simulink model "test_mdl"  (R2018a)
settings: Solver=VariableStepAuto  StartTime=0.0  StopTime=10.0  RelTol=1e-3
(part 5 of 8)

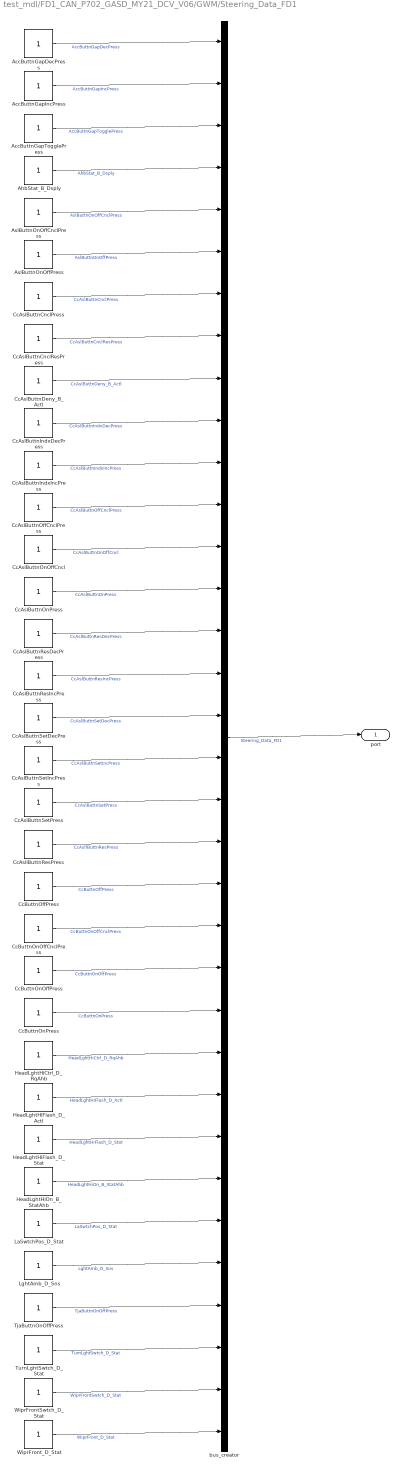
== system test_mdl/FD1_CAN_P702_GASD_MY21_DCV_V06/GWM/Steering_Data_FD1 ==
  AccButtnGapDecPress : Constant
  AccButtnGapIncPress : Constant
  AccButtnGapTogglePress : Constant
  AhbStat_B_Dsply : Constant
  AslButtnOnOffCnclPress : Constant
  AslButtnOnOffPress : Constant
  CcAslButtnCnclPress : Constant
  CcAslButtnCnclResPress : Constant
  CcAslButtnDeny_B_Actl : Constant
  CcAslButtnIndxDecPress : Constant
  CcAslButtnIndxIncPress : Constant
  CcAslButtnOffCnclPress : Constant
  CcAslButtnOnOffCncl : Constant
  CcAslButtnOnPress : Constant
  CcAslButtnResDecPress : Constant
  CcAslButtnResIncPress : Constant
  CcAslButtnSetDecPress : Constant
  CcAslButtnSetIncPress : Constant
  CcAslButtnSetPress : Constant
  CcAsllButtnResPress : Constant
  CcButtnOffPress : Constant
  CcButtnOnOffCnclPress : Constant
  CcButtnOnOffPress : Constant
  CcButtnOnPress : Constant
  HeadLghtHiCtrl_D_RqAhb : Constant
  HeadLghtHiFlash_D_Actl : Constant
  HeadLghtHiFlash_D_Stat : Constant
  HeadLghtHiOn_B_StatAhb : Constant
  LaSwtchPos_D_Stat : Constant
  LghtAmb_D_Sns : Constant
  TjaButtnOnOffPress : Constant
  TurnLghtSwtch_D_Stat : Constant
  WiprFrontSwtch_D_Stat : Constant
  WiprFront_D_Stat : Constant
  bus_creator : BusCreator  Inputs=34
  port : Outport
  wires:
  bus_creator/1 -> port/1  "Steering_Data_FD1"
  AccButtnGapDecPress/1 -> bus_creator/1  "AccButtnGapDecPress"
  AccButtnGapIncPress/1 -> bus_creator/2  "AccButtnGapIncPress"
  AccButtnGapTogglePress/1 -> bus_creator/3  "AccButtnGapTogglePress"
  AhbStat_B_Dsply/1 -> bus_creator/4  "AhbStat_B_Dsply"
  AslButtnOnOffCnclPress/1 -> bus_creator/5  "AslButtnOnOffCnclPress"
  AslButtnOnOffPress/1 -> bus_creator/6  "AslButtnOnOffPress"
  CcAslButtnCnclPress/1 -> bus_creator/7  "CcAslButtnCnclPress"
  CcAslButtnCnclResPress/1 -> bus_creator/8  "CcAslButtnCnclResPress"
  CcAslButtnDeny_B_Actl/1 -> bus_creator/9  "CcAslButtnDeny_B_Actl"
  CcAslButtnIndxDecPress/1 -> bus_creator/10  "CcAslButtnIndxDecPress"
  CcAslButtnIndxIncPress/1 -> bus_creator/11  "CcAslButtnIndxIncPress"
  CcAslButtnOffCnclPress/1 -> bus_creator/12  "CcAslButtnOffCnclPress"
  CcAslButtnOnOffCncl/1 -> bus_creator/13  "CcAslButtnOnOffCncl"
  CcAslButtnOnPress/1 -> bus_creator/14  "CcAslButtnOnPress"
  CcAslButtnResDecPress/1 -> bus_creator/15  "CcAslButtnResDecPress"
  CcAslButtnResIncPress/1 -> bus_creator/16  "CcAslButtnResIncPress"
  CcAslButtnSetDecPress/1 -> bus_creator/17  "CcAslButtnSetDecPress"
  CcAslButtnSetIncPress/1 -> bus_creator/18  "CcAslButtnSetIncPress"
  CcAslButtnSetPress/1 -> bus_creator/19  "CcAslButtnSetPress"
  CcAsllButtnResPress/1 -> bus_creator/20  "CcAsllButtnResPress"
  CcButtnOffPress/1 -> bus_creator/21  "CcButtnOffPress"
  CcButtnOnOffCnclPress/1 -> bus_creator/22  "CcButtnOnOffCnclPress"
  CcButtnOnOffPress/1 -> bus_creator/23  "CcButtnOnOffPress"
  CcButtnOnPress/1 -> bus_creator/24  "CcButtnOnPress"
  HeadLghtHiCtrl_D_RqAhb/1 -> bus_creator/25  "HeadLghtHiCtrl_D_RqAhb"
  HeadLghtHiFlash_D_Actl/1 -> bus_creator/26  "HeadLghtHiFlash_D_Actl"
  HeadLghtHiFlash_D_Stat/1 -> bus_creator/27  "HeadLghtHiFlash_D_Stat"
  HeadLghtHiOn_B_StatAhb/1 -> bus_creator/28  "HeadLghtHiOn_B_StatAhb"
  LaSwtchPos_D_Stat/1 -> bus_creator/29  "LaSwtchPos_D_Stat"
  LghtAmb_D_Sns/1 -> bus_creator/30  "LghtAmb_D_Sns"
  TjaButtnOnOffPress/1 -> bus_creator/31  "TjaButtnOnOffPress"
  TurnLghtSwtch_D_Stat/1 -> bus_creator/32  "TurnLghtSwtch_D_Stat"
  WiprFrontSwtch_D_Stat/1 -> bus_creator/33  "WiprFrontSwtch_D_Stat"
  WiprFront_D_Stat/1 -> bus_creator/34  "WiprFront_D_Stat"

== system test_mdl/FD1_CAN_P702_GASD_MY21_DCV_V06/GWM/Steering_Wheel_Data2_FD1 ==
  SelDrvMdeDec_B_RqDrv : Constant
  SelDrvMdeInc_B_RqDrv : Constant
  SelDrvMdeSwtch_D_Stat4 : Constant
  SteEffortInc_B_RqDrv : Constant
  SteWhlSwtchBack_B_Stat : Constant
  SteWhlSwtchDown_B_Stat : Constant
  SteWhlSwtchHome_B_Stat : Constant
  SteWhlSwtchHud_B_Stat : Constant
  SteWhlSwtchInfo_B_Stat : Constant
  SteWhlSwtchIod_B_Stat : Constant
  SteWhlSwtchLeft_B_Stat : Constant
  SteWhlSwtchMed_B_Stat : Constant
  SteWhlSwtchMenu_B_Stat : Constant
  SteWhlSwtchNav_B_Stat : Constant
  SteWhlSwtchOk_B_Stat : Constant
  SteWhlSwtchPhon_B_Stat : Constant
  SteWhlSwtchRght_B_Stat : Constant
  SteWhlSwtchSet_B_Stat : Constant
  SteWhlSwtchUp_B_Stat : Constant
  SteWhlSwtchView_B_Stat : Constant
  SuspDampInc_B_RqDrv : Constant
  bus_creator : BusCreator  Inputs=21
  port : Outport
  wires:
  bus_creator/1 -> port/1  "Steering_Wheel_Data2_FD1"
  SelDrvMdeDec_B_RqDrv/1 -> bus_creator/1  "SelDrvMdeDec_B_RqDrv"
  SelDrvMdeInc_B_RqDrv/1 -> bus_creator/2  "SelDrvMdeInc_B_RqDrv"
  SelDrvMdeSwtch_D_Stat4/1 -> bus_creator/3  "SelDrvMdeSwtch_D_Stat4"
  SteEffortInc_B_RqDrv/1 -> bus_creator/4  "SteEffortInc_B_RqDrv"
  SteWhlSwtchBack_B_Stat/1 -> bus_creator/5  "SteWhlSwtchBack_B_Stat"
  SteWhlSwtchDown_B_Stat/1 -> bus_creator/6  "SteWhlSwtchDown_B_Stat"
  SteWhlSwtchHome_B_Stat/1 -> bus_creator/7  "SteWhlSwtchHome_B_Stat"
  SteWhlSwtchHud_B_Stat/1 -> bus_creator/8  "SteWhlSwtchHud_B_Stat"
  SteWhlSwtchInfo_B_Stat/1 -> bus_creator/9  "SteWhlSwtchInfo_B_Stat"
  SteWhlSwtchIod_B_Stat/1 -> bus_creator/10  "SteWhlSwtchIod_B_Stat"
  SteWhlSwtchLeft_B_Stat/1 -> bus_creator/11  "SteWhlSwtchLeft_B_Stat"
  SteWhlSwtchMed_B_Stat/1 -> bus_creator/12  "SteWhlSwtchMed_B_Stat"
  SteWhlSwtchMenu_B_Stat/1 -> bus_creator/13  "SteWhlSwtchMenu_B_Stat"
  SteWhlSwtchNav_B_Stat/1 -> bus_creator/14  "SteWhlSwtchNav_B_Stat"
  SteWhlSwtchOk_B_Stat/1 -> bus_creator/15  "SteWhlSwtchOk_B_Stat"
  SteWhlSwtchPhon_B_Stat/1 -> bus_creator/16  "SteWhlSwtchPhon_B_Stat"
  SteWhlSwtchRght_B_Stat/1 -> bus_creator/17  "SteWhlSwtchRght_B_Stat"
  SteWhlSwtchSet_B_Stat/1 -> bus_creator/18  "SteWhlSwtchSet_B_Stat"
  SteWhlSwtchUp_B_Stat/1 -> bus_creator/19  "SteWhlSwtchUp_B_Stat"
  SteWhlSwtchView_B_Stat/1 -> bus_creator/20  "SteWhlSwtchView_B_Stat"
  SuspDampInc_B_RqDrv/1 -> bus_creator/21  "SuspDampInc_B_RqDrv"

== system test_mdl/FD1_CAN_P702_GASD_MY21_DCV_V06/GWM/TCU_Send_Signals_FD1 ==
  EmgcyCallMute_D_Stat : Constant
  OfbChrgSetSync_D_Rq : Constant
  TelematicsSrvc_D_St : Constant
  bus_creator : BusCreator  Inputs=3
  port : Outport
  wires:
  bus_creator/1 -> port/1  "TCU_Send_Signals_FD1"
  EmgcyCallMute_D_Stat/1 -> bus_creator/1  "EmgcyCallMute_D_Stat"
  OfbChrgSetSync_D_Rq/1 -> bus_creator/2  "OfbChrgSetSync_D_Rq"
  TelematicsSrvc_D_St/1 -> bus_creator/3  "TelematicsSrvc_D_St"

== system test_mdl/FD1_CAN_P702_GASD_MY21_DCV_V06/GWM/TesterPhysicalReqVDM_FD1 ==
  TesterPhysicalReqVDM : Constant
  bus_creator : BusCreator  Inputs=1
  port : Outport
  wires:
  bus_creator/1 -> port/1  "TesterPhysicalReqVDM_FD1"
  TesterPhysicalReqVDM/1 -> bus_creator/1  "TesterPhysicalReqVDM"

== system test_mdl/FD1_CAN_P702_GASD_MY21_DCV_V06/GWM/TesterPhysicalResGWM_FD1 ==
  TesterPhysicalResGWM_F1 : Constant
  bus_creator : BusCreator  Inputs=1
  port : Outport
  wires:
  bus_creator/1 -> port/1  "TesterPhysicalResGWM_FD1"
  TesterPhysicalResGWM_F1/1 -> bus_creator/1  "TesterPhysicalResGWM_F1"

== system test_mdl/FD1_CAN_P702_GASD_MY21_DCV_V06/GWM/Tire_Pressure_Data_FD1 ==
  Tire_Press_LF_Data : Constant
  Tire_Press_LR_OLR_Data : Constant
  Tire_Press_RF_Data : Constant
  Tire_Press_RR_ORR_Data : Constant
  bus_creator : BusCreator  Inputs=4
  port : Outport
  wires:
  bus_creator/1 -> port/1  "Tire_Pressure_Data_FD1"
  Tire_Press_LF_Data/1 -> bus_creator/1  "Tire_Press_LF_Data"
  Tire_Press_LR_OLR_Data/1 -> bus_creator/2  "Tire_Press_LR_OLR_Data"
  Tire_Press_RF_Data/1 -> bus_creator/3  "Tire_Press_RF_Data"
  Tire_Press_RR_ORR_Data/1 -> bus_creator/4  "Tire_Press_RR_ORR_Data"

== system test_mdl/FD1_CAN_P702_GASD_MY21_DCV_V06/GWM/TrailerAid_Data3_FD1 ==
  TrlrAidEnbl_D2_Rq : Constant
  TrlrAidSetup_D2_Rq : Constant
  TrlrAnOffstDir_D_Mem : Constant
  TrlrAnOffst_An_Mem : Constant
  TrlrAxleToBmpr_L_Actl : Constant
  TrlrBallToBmpr_L_Actl : Constant
  TrlrIdType_D_Stat : Constant
  TrlrId_No_Actl : Constant
  TrlrRvrseCancl_B_Rq : Constant
  TrlrTrgtOffst_L_Actl : Constant
  TrlrTrgtPtrnId_No_Mem : Constant
  TrlrTrgtToBmpr_L_Actl : Constant
  bus_creator : BusCreator  Inputs=12
  port : Outport
  wires:
  bus_creator/1 -> port/1  "TrailerAid_Data3_FD1"
  TrlrAidEnbl_D2_Rq/1 -> bus_creator/1  "TrlrAidEnbl_D2_Rq"
  TrlrAidSetup_D2_Rq/1 -> bus_creator/2  "TrlrAidSetup_D2_Rq"
  TrlrAnOffstDir_D_Mem/1 -> bus_creator/3  "TrlrAnOffstDir_D_Mem"
  TrlrAnOffst_An_Mem/1 -> bus_creator/4  "TrlrAnOffst_An_Mem"
  TrlrAxleToBmpr_L_Actl/1 -> bus_creator/5  "TrlrAxleToBmpr_L_Actl"
  TrlrBallToBmpr_L_Actl/1 -> bus_creator/6  "TrlrBallToBmpr_L_Actl"
  TrlrIdType_D_Stat/1 -> bus_creator/7  "TrlrIdType_D_Stat"
  TrlrId_No_Actl/1 -> bus_creator/8  "TrlrId_No_Actl"
  TrlrRvrseCancl_B_Rq/1 -> bus_creator/9  "TrlrRvrseCancl_B_Rq"
  TrlrTrgtOffst_L_Actl/1 -> bus_creator/10  "TrlrTrgtOffst_L_Actl"
  TrlrTrgtPtrnId_No_Mem/1 -> bus_creator/11  "TrlrTrgtPtrnId_No_Mem"
  TrlrTrgtToBmpr_L_Actl/1 -> bus_creator/12  "TrlrTrgtToBmpr_L_Actl"

== system test_mdl/FD1_CAN_P702_GASD_MY21_DCV_V06/GWM/TrailerAid_Data_FD1 ==
  TrailCtlSwtch_B_Stat2 : Constant
  TrlBrkInitOut_D_Rq : Constant
  bus_creator : BusCreator  Inputs=2
  port : Outport
  wires:
  bus_creator/1 -> port/1  "TrailerAid_Data_FD1"
  TrailCtlSwtch_B_Stat2/1 -> bus_creator/1  "TrailCtlSwtch_B_Stat2"
  TrlBrkInitOut_D_Rq/1 -> bus_creator/2  "TrlBrkInitOut_D_Rq"

== system test_mdl/FD1_CAN_P702_GASD_MY21_DCV_V06/GWM/TrailerAid_Stat1_FD1 ==
  TrlrSnsId_No_Actl : Constant
  bus_creator : BusCreator  Inputs=1
  port : Outport
  wires:
  bus_creator/1 -> port/1  "TrailerAid_Stat1_FD1"
  TrlrSnsId_No_Actl/1 -> bus_creator/1  "TrlrSnsId_No_Actl"

== system test_mdl/FD1_CAN_P702_GASD_MY21_DCV_V06/GWM/TrailerAid_Stat2_FD1 ==
  TrlrHitYaw_AnRate_Actl : Constant
  TrlrHitchYaw_An_Actl : Constant
  TrlrHitchYaw_D_Stat : Constant
  TrlrYawWActl_D_Qf : Constant
  TrlrYaw_W_Actl : Constant
  bus_creator : BusCreator  Inputs=5
  port : Outport
  wires:
  bus_creator/1 -> port/1  "TrailerAid_Stat2_FD1"
  TrlrHitYaw_AnRate_Actl/1 -> bus_creator/1  "TrlrHitYaw_AnRate_Actl"
  TrlrHitchYaw_An_Actl/1 -> bus_creator/2  "TrlrHitchYaw_An_Actl"
  TrlrHitchYaw_D_Stat/1 -> bus_creator/3  "TrlrHitchYaw_D_Stat"
  TrlrYawWActl_D_Qf/1 -> bus_creator/4  "TrlrYawWActl_D_Qf"
  TrlrYaw_W_Actl/1 -> bus_creator/5  "TrlrYaw_W_Actl"

== system test_mdl/FD1_CAN_P702_GASD_MY21_DCV_V06/GWM/TrailerBrakeInfo_FD1 ==
  StopLamp_B_RqTrlrBrk : Constant
  TrlBrkInitOut_D_Stat : Constant
  TrlrBrkActCirct_B_Falt : Constant
  TrlrBrkActCnnct_B_Actl : Constant
  TrlrBrkCtl_B_Falt : Constant
  TrlrBrkDcnnt_B_Actl : Constant
  TrlrBrkDsply_B_Rq : Constant
  TrlrBrkGain_No_Actl : Constant
  TrlrBrkMde_D_Actl : Constant
  TrlrBrkOut_No_Dsply : Constant
  bus_creator : BusCreator  Inputs=10
  port : Outport
  wires:
  bus_creator/1 -> port/1  "TrailerBrakeInfo_FD1"
  StopLamp_B_RqTrlrBrk/1 -> bus_creator/1  "StopLamp_B_RqTrlrBrk"
  TrlBrkInitOut_D_Stat/1 -> bus_creator/2  "TrlBrkInitOut_D_Stat"
  TrlrBrkActCirct_B_Falt/1 -> bus_creator/3  "TrlrBrkActCirct_B_Falt"
  TrlrBrkActCnnct_B_Actl/1 -> bus_creator/4  "TrlrBrkActCnnct_B_Actl"
  TrlrBrkCtl_B_Falt/1 -> bus_creator/5  "TrlrBrkCtl_B_Falt"
  TrlrBrkDcnnt_B_Actl/1 -> bus_creator/6  "TrlrBrkDcnnt_B_Actl"
  TrlrBrkDsply_B_Rq/1 -> bus_creator/7  "TrlrBrkDsply_B_Rq"
  TrlrBrkGain_No_Actl/1 -> bus_creator/8  "TrlrBrkGain_No_Actl"
  TrlrBrkMde_D_Actl/1 -> bus_creator/9  "TrlrBrkMde_D_Actl"
  TrlrBrkOut_No_Dsply/1 -> bus_creator/10  "TrlrBrkOut_No_Dsply"

== system test_mdl/FD1_CAN_P702_GASD_MY21_DCV_V06/GWM/TrailerInfo_2_FD1 ==
  TrlrAidCtl_U_RqDrv : Constant
  TrlrAidSwtch_D_RqDrv : Constant
  bus_creator : BusCreator  Inputs=2
  port : Outport
  wires:
  bus_creator/1 -> port/1  "TrailerInfo_2_FD1"
  TrlrAidCtl_U_RqDrv/1 -> bus_creator/1  "TrlrAidCtl_U_RqDrv"
  TrlrAidSwtch_D_RqDrv/1 -> bus_creator/2  "TrlrAidSwtch_D_RqDrv"

== system test_mdl/FD1_CAN_P702_GASD_MY21_DCV_V06/GWM/TrailerInfo_FD1 ==
  ParkLampTrlrOut_B_Stat : Constant
  StopLampTrlrOut_B_Stat : Constant
  TrlrBattChrg_D_Stat : Constant
  TrlrLampCnnct_B_Actl : Constant
  TrlrLampCtl_D_Stat : Constant
  TurnLampTrlrRl_B_Stat : Constant
  TurnLampTrlrRr_B_Stat : Constant
  bus_creator : BusCreator  Inputs=7
  port : Outport
  wires:
  bus_creator/1 -> port/1  "TrailerInfo_FD1"
  ParkLampTrlrOut_B_Stat/1 -> bus_creator/1  "ParkLampTrlrOut_B_Stat"
  StopLampTrlrOut_B_Stat/1 -> bus_creator/2  "StopLampTrlrOut_B_Stat"
  TrlrBattChrg_D_Stat/1 -> bus_creator/3  "TrlrBattChrg_D_Stat"
  TrlrLampCnnct_B_Actl/1 -> bus_creator/4  "TrlrLampCnnct_B_Actl"
  TrlrLampCtl_D_Stat/1 -> bus_creator/5  "TrlrLampCtl_D_Stat"
  TurnLampTrlrRl_B_Stat/1 -> bus_creator/6  "TurnLampTrlrRl_B_Stat"
  TurnLampTrlrRr_B_Stat/1 -> bus_creator/7  "TurnLampTrlrRr_B_Stat"

== system test_mdl/FD1_CAN_P702_GASD_MY21_DCV_V06/GWM/Voltage_Power_Data2_FD1 ==
  CoolFanDcdc_D_Rq : Constant
  DcdcClntFlw_D_Rq : Constant
  bus_creator : BusCreator  Inputs=2
  port : Outport
  wires:
  bus_creator/1 -> port/1  "Voltage_Power_Data2_FD1"
  CoolFanDcdc_D_Rq/1 -> bus_creator/1  "CoolFanDcdc_D_Rq"
  DcdcClntFlw_D_Rq/1 -> bus_creator/2  "DcdcClntFlw_D_Rq"

== system test_mdl/FD1_CAN_P702_GASD_MY21_DCV_V06/GWM/Yaw_Data_FD1 ==
  VehRolWActl_D_Qf : Constant
  VehRol_W_Actl : Constant
  VehRollYawW_No_Cs : Constant
  VehRollYaw_No_Cnt : Constant
  VehYawWActl_D_Qf : Constant
  VehYaw_W_Actl : Constant
  bus_creator : BusCreator  Inputs=6
  port : Outport
  wires:
  bus_creator/1 -> port/1  "Yaw_Data_FD1"
  VehRolWActl_D_Qf/1 -> bus_creator/1  "VehRolWActl_D_Qf"
  VehRol_W_Actl/1 -> bus_creator/2  "VehRol_W_Actl"
  VehRollYawW_No_Cs/1 -> bus_creator/3  "VehRollYawW_No_Cs"
  VehRollYaw_No_Cnt/1 -> bus_creator/4  "VehRollYaw_No_Cnt"
  VehYawWActl_D_Qf/1 -> bus_creator/5  "VehYawWActl_D_Qf"
  VehYaw_W_Actl/1 -> bus_creator/6  "VehYaw_W_Actl"

== system test_mdl/FD1_CAN_P702_GASD_MY21_DCV_V06/IPMA_ADAS/ACCDATA ==
  AccAutoResum_D_Rq : Constant
  AccBrkDecel_B_Rq : Constant
  AccBrkPrchg_B_Rq : Constant
  AccBrkPrkEl_B_Rq : Constant
  AccBrkPulse_B_Rq : Constant
  AccBrkTot_A_Rq : Constant
  AccCancl_B_Rq : Constant
  AccDeny_B_Rq : Constant
  AccPrpl_A_Pred : Constant
  AccPrpl_A_Rq : Constant
  AccResumEnbl_B_Rq : Constant
  AccStopStat_B_Rq : Constant
  AccVeh_V_Trg : Constant
  CmbbDeny_B_Actl : Constant
  CmbbEngTqMn_B_Rq : Constant
  CmbbOvrrd_B_RqDrv : Constant
  Cmbb_B_Enbl : Constant
  bus_creator : BusCreator  Inputs=17
  port : Outport
  wires:
  bus_creator/1 -> port/1  "ACCDATA"
  AccAutoResum_D_Rq/1 -> bus_creator/1  "AccAutoResum_D_Rq"
  AccBrkDecel_B_Rq/1 -> bus_creator/2  "AccBrkDecel_B_Rq"
  AccBrkPrchg_B_Rq/1 -> bus_creator/3  "AccBrkPrchg_B_Rq"
  AccBrkPrkEl_B_Rq/1 -> bus_creator/4  "AccBrkPrkEl_B_Rq"
  AccBrkPulse_B_Rq/1 -> bus_creator/5  "AccBrkPulse_B_Rq"
  AccBrkTot_A_Rq/1 -> bus_creator/6  "AccBrkTot_A_Rq"
  AccCancl_B_Rq/1 -> bus_creator/7  "AccCancl_B_Rq"
  AccDeny_B_Rq/1 -> bus_creator/8  "AccDeny_B_Rq"
  AccPrpl_A_Pred/1 -> bus_creator/9  "AccPrpl_A_Pred"
  AccPrpl_A_Rq/1 -> bus_creator/10  "AccPrpl_A_Rq"
  AccResumEnbl_B_Rq/1 -> bus_creator/11  "AccResumEnbl_B_Rq"
  AccStopStat_B_Rq/1 -> bus_creator/12  "AccStopStat_B_Rq"
  AccVeh_V_Trg/1 -> bus_creator/13  "AccVeh_V_Trg"
  CmbbDeny_B_Actl/1 -> bus_creator/14  "CmbbDeny_B_Actl"
  CmbbEngTqMn_B_Rq/1 -> bus_creator/15  "CmbbEngTqMn_B_Rq"
  CmbbOvrrd_B_RqDrv/1 -> bus_creator/16  "CmbbOvrrd_B_RqDrv"
  Cmbb_B_Enbl/1 -> bus_creator/17  "Cmbb_B_Enbl"

== system test_mdl/FD1_CAN_P702_GASD_MY21_DCV_V06/IPMA_ADAS/ACCDATA_2 ==
  CmbbBaSens_D_Rq : Constant
  CmbbBrkDecel_A_Rq : Constant
  CmbbBrkDecel_B_Rq : Constant
  CmbbBrkDecel_No_Cnt : Constant
  CmbbBrkDecel_No_Cs : Constant
  CmbbBrkPrchg_D_Rq : Constant
  HudBlk1_B_Rq : Constant
  HudBlk2_B_Rq : Constant
  HudBlk3_B_Rq : Constant
  HudDsplyIntns_No_Actl : Constant
  HudFlashRate_D_Actl : Constant
  bus_creator : BusCreator  Inputs=11
  port : Outport
  wires:
  bus_creator/1 -> port/1  "ACCDATA_2"
  CmbbBaSens_D_Rq/1 -> bus_creator/1  "CmbbBaSens_D_Rq"
  CmbbBrkDecel_A_Rq/1 -> bus_creator/2  "CmbbBrkDecel_A_Rq"
  CmbbBrkDecel_B_Rq/1 -> bus_creator/3  "CmbbBrkDecel_B_Rq"
  CmbbBrkDecel_No_Cnt/1 -> bus_creator/4  "CmbbBrkDecel_No_Cnt"
  CmbbBrkDecel_No_Cs/1 -> bus_creator/5  "CmbbBrkDecel_No_Cs"
  CmbbBrkPrchg_D_Rq/1 -> bus_creator/6  "CmbbBrkPrchg_D_Rq"
  HudBlk1_B_Rq/1 -> bus_creator/7  "HudBlk1_B_Rq"
  HudBlk2_B_Rq/1 -> bus_creator/8  "HudBlk2_B_Rq"
  HudBlk3_B_Rq/1 -> bus_creator/9  "HudBlk3_B_Rq"
  HudDsplyIntns_No_Actl/1 -> bus_creator/10  "HudDsplyIntns_No_Actl"
  HudFlashRate_D_Actl/1 -> bus_creator/11  "HudFlashRate_D_Actl"

== system test_mdl/FD1_CAN_P702_GASD_MY21_DCV_V06/IPMA_ADAS/ACCDATA_3 ==
  AccFllwMde_B_Dsply : Constant
  AccMemEnbl_B_RqDrv : Constant
  AccMsgTxt_D2_Rq : Constant
  AccStopMde_B_Dsply : Constant
  AccStopRes_B_Dsply : Constant
  AccStopStat_D_Dsply : Constant
  AccTGap_B_Dsply : Constant
  AccTGap_D_Dsply : Constant
  AccTrgDist2_D_Dsply : Constant
  AccWarn_D_Dsply : Constant
  CadsAlignIncplt_B_Actl : Constant
  CadsRadrBlck_B_Actl : Constant
  CmbbPostEvnt_B_Dsply : Constant
  FcwAudioWarn_B_Rq : Constant
  FcwDeny_B_Dsply : Constant
  FcwMemSens_D_Actl : Constant
  FcwMemStat_B_Actl : Constant
  FcwMsgTxt_D_Rq : Constant
  FcwVisblWarn_B_Rq : Constant
  FdaMem_B_Stat : Constant
  HaDsply_No_Cnt : Constant
  HaDsply_No_Cs : Constant
  IaccLamp_D_Rq : Constant
  TjaMsgTxt_D_Dsply : Constant
  TjaWarn_D_Rq : Constant
  Tja_D_Stat : Constant
  bus_creator : BusCreator  Inputs=26
  port : Outport
  wires:
  bus_creator/1 -> port/1  "ACCDATA_3"
  AccFllwMde_B_Dsply/1 -> bus_creator/1  "AccFllwMde_B_Dsply"
  AccMemEnbl_B_RqDrv/1 -> bus_creator/2  "AccMemEnbl_B_RqDrv"
  AccMsgTxt_D2_Rq/1 -> bus_creator/3  "AccMsgTxt_D2_Rq"
  AccStopMde_B_Dsply/1 -> bus_creator/4  "AccStopMde_B_Dsply"
  AccStopRes_B_Dsply/1 -> bus_creator/5  "AccStopRes_B_Dsply"
  AccStopStat_D_Dsply/1 -> bus_creator/6  "AccStopStat_D_Dsply"
  AccTGap_B_Dsply/1 -> bus_creator/7  "AccTGap_B_Dsply"
  AccTGap_D_Dsply/1 -> bus_creator/8  "AccTGap_D_Dsply"
  AccTrgDist2_D_Dsply/1 -> bus_creator/9  "AccTrgDist2_D_Dsply"
  AccWarn_D_Dsply/1 -> bus_creator/10  "AccWarn_D_Dsply"
  CadsAlignIncplt_B_Actl/1 -> bus_creator/11  "CadsAlignIncplt_B_Actl"
  CadsRadrBlck_B_Actl/1 -> bus_creator/12  "CadsRadrBlck_B_Actl"
  CmbbPostEvnt_B_Dsply/1 -> bus_creator/13  "CmbbPostEvnt_B_Dsply"
  FcwAudioWarn_B_Rq/1 -> bus_creator/14  "FcwAudioWarn_B_Rq"
  FcwDeny_B_Dsply/1 -> bus_creator/15  "FcwDeny_B_Dsply"
  FcwMemSens_D_Actl/1 -> bus_creator/16  "FcwMemSens_D_Actl"
  FcwMemStat_B_Actl/1 -> bus_creator/17  "FcwMemStat_B_Actl"
  FcwMsgTxt_D_Rq/1 -> bus_creator/18  "FcwMsgTxt_D_Rq"
  FcwVisblWarn_B_Rq/1 -> bus_creator/19  "FcwVisblWarn_B_Rq"
  FdaMem_B_Stat/1 -> bus_creator/20  "FdaMem_B_Stat"
  HaDsply_No_Cnt/1 -> bus_creator/21  "HaDsply_No_Cnt"
  HaDsply_No_Cs/1 -> bus_creator/22  "HaDsply_No_Cs"
  IaccLamp_D_Rq/1 -> bus_creator/23  "IaccLamp_D_Rq"
  TjaMsgTxt_D_Dsply/1 -> bus_creator/24  "TjaMsgTxt_D_Dsply"
  TjaWarn_D_Rq/1 -> bus_creator/25  "TjaWarn_D_Rq"
  Tja_D_Stat/1 -> bus_creator/26  "Tja_D_Stat"

== system test_mdl/FD1_CAN_P702_GASD_MY21_DCV_V06/IPMA_ADAS/AutoDriveBeam_Data1 ==
  AdbBrdr1CritLeft_T_Stat : Constant
  AdbBrdr1CritRigh_T_Stat : Constant
  AdbBrdr1DistLeft_D_Stat : Constant
  AdbBrdr1DistRigh_D_Stat : Constant
  AdbBrdr1Left_An_Rq : Constant
  AdbBrdr1Low_An_Rq : Constant
  AdbBrdr1Right_An_Rq : Constant
  AdbBrdr1Up_An_Rq : Constant
  AdbIntns1_D_Rq : Constant
  AdbMde1_D_Rq : Constant
  bus_creator : BusCreator  Inputs=10
  port : Outport
  wires:
  bus_creator/1 -> port/1  "AutoDriveBeam_Data1"
  AdbBrdr1CritLeft_T_Stat/1 -> bus_creator/1  "AdbBrdr1CritLeft_T_Stat"
  AdbBrdr1CritRigh_T_Stat/1 -> bus_creator/2  "AdbBrdr1CritRigh_T_Stat"
  AdbBrdr1DistLeft_D_Stat/1 -> bus_creator/3  "AdbBrdr1DistLeft_D_Stat"
  AdbBrdr1DistRigh_D_Stat/1 -> bus_creator/4  "AdbBrdr1DistRigh_D_Stat"
  AdbBrdr1Left_An_Rq/1 -> bus_creator/5  "AdbBrdr1Left_An_Rq"
  AdbBrdr1Low_An_Rq/1 -> bus_creator/6  "AdbBrdr1Low_An_Rq"
  AdbBrdr1Right_An_Rq/1 -> bus_creator/7  "AdbBrdr1Right_An_Rq"
  AdbBrdr1Up_An_Rq/1 -> bus_creator/8  "AdbBrdr1Up_An_Rq"
  AdbIntns1_D_Rq/1 -> bus_creator/9  "AdbIntns1_D_Rq"
  AdbMde1_D_Rq/1 -> bus_creator/10  "AdbMde1_D_Rq"

== system test_mdl/FD1_CAN_P702_GASD_MY21_DCV_V06/IPMA_ADAS/AutoDriveBeam_Data2 ==
  AdbBrdr2CritLeft_T_Stat : Constant
  AdbBrdr2CritRigh_T_Stat : Constant
  AdbBrdr2DistLeft_D_Stat : Constant
  AdbBrdr2DistRigh_D_Stat : Constant
  AdbBrdr2Left_An_Rq : Constant
  AdbBrdr2Low_An_Rq : Constant
  AdbBrdr2Right_An_Rq : Constant
  AdbBrdr2Up_An_Rq : Constant
  AdbIntns2_D_Rq : Constant
  AdbMde2_D_Rq : Constant
  bus_creator : BusCreator  Inputs=10
  port : Outport
  wires:
  bus_creator/1 -> port/1  "AutoDriveBeam_Data2"
  AdbBrdr2CritLeft_T_Stat/1 -> bus_creator/1  "AdbBrdr2CritLeft_T_Stat"
  AdbBrdr2CritRigh_T_Stat/1 -> bus_creator/2  "AdbBrdr2CritRigh_T_Stat"
  AdbBrdr2DistLeft_D_Stat/1 -> bus_creator/3  "AdbBrdr2DistLeft_D_Stat"
  AdbBrdr2DistRigh_D_Stat/1 -> bus_creator/4  "AdbBrdr2DistRigh_D_Stat"
  AdbBrdr2Left_An_Rq/1 -> bus_creator/5  "AdbBrdr2Left_An_Rq"
  AdbBrdr2Low_An_Rq/1 -> bus_creator/6  "AdbBrdr2Low_An_Rq"
  AdbBrdr2Right_An_Rq/1 -> bus_creator/7  "AdbBrdr2Right_An_Rq"
  AdbBrdr2Up_An_Rq/1 -> bus_creator/8  "AdbBrdr2Up_An_Rq"
  AdbIntns2_D_Rq/1 -> bus_creator/9  "AdbIntns2_D_Rq"
  AdbMde2_D_Rq/1 -> bus_creator/10  "AdbMde2_D_Rq"

== system test_mdl/FD1_CAN_P702_GASD_MY21_DCV_V06/IPMA_ADAS/AutoDriveBeam_Data3 ==
  AdbBrdr3CritLeft_T_Stat : Constant
  AdbBrdr3CritRigh_T_Stat : Constant
  AdbBrdr3DistLeft_D_Stat : Constant
  AdbBrdr3DistRigh_D_Stat : Constant
  AdbBrdr3Left_An_Rq : Constant
  AdbBrdr3Low_An_Rq : Constant
  AdbBrdr3Right_An_Rq : Constant
  AdbBrdr3Up_An_Rq : Constant
  AdbIntns3_D_Rq : Constant
  AdbMde3_D_Rq : Constant
  bus_creator : BusCreator  Inputs=10
  port : Outport
  wires:
  bus_creator/1 -> port/1  "AutoDriveBeam_Data3"
  AdbBrdr3CritLeft_T_Stat/1 -> bus_creator/1  "AdbBrdr3CritLeft_T_Stat"
  AdbBrdr3CritRigh_T_Stat/1 -> bus_creator/2  "AdbBrdr3CritRigh_T_Stat"
  AdbBrdr3DistLeft_D_Stat/1 -> bus_creator/3  "AdbBrdr3DistLeft_D_Stat"
  AdbBrdr3DistRigh_D_Stat/1 -> bus_creator/4  "AdbBrdr3DistRigh_D_Stat"
  AdbBrdr3Left_An_Rq/1 -> bus_creator/5  "AdbBrdr3Left_An_Rq"
  AdbBrdr3Low_An_Rq/1 -> bus_creator/6  "AdbBrdr3Low_An_Rq"
  AdbBrdr3Right_An_Rq/1 -> bus_creator/7  "AdbBrdr3Right_An_Rq"
  AdbBrdr3Up_An_Rq/1 -> bus_creator/8  "AdbBrdr3Up_An_Rq"
  AdbIntns3_D_Rq/1 -> bus_creator/9  "AdbIntns3_D_Rq"
  AdbMde3_D_Rq/1 -> bus_creator/10  "AdbMde3_D_Rq"

== system test_mdl/FD1_CAN_P702_GASD_MY21_DCV_V06/IPMA_ADAS/Bndry_Alert_L_Data ==
  BalrChimeLeft_D_Rq : Constant
  BalrLckLeft_B_Stat : Constant
  BalrLeft_D_Stat : Constant
  BalrMdeLeft_D_Stat : Constant
  BalrMdeSelLeft_B_Stat : Constant
  BalrSnsLeft_D_Falt : Constant
  BalrWndwLeft_B_Stat : Constant
  CamraRearOn_B_RqBalrl : Constant
  DrLckActv_B_RqBalrl : Constant
  DrLckCnt_No_ActlBalrl : Constant
  WndwDrvRear_D_RqBalrl : Constant
  WndwDrv_D_RqBalrl : Constant
  WndwPsngrRear_D_RqBalrl : Constant
  WndwPsngr_D_RqBalrl : Constant
  bus_creator : BusCreator  Inputs=14
  port : Outport
  wires:
  bus_creator/1 -> port/1  "Bndry_Alert_L_Data"
  BalrChimeLeft_D_Rq/1 -> bus_creator/1  "BalrChimeLeft_D_Rq"
  BalrLckLeft_B_Stat/1 -> bus_creator/2  "BalrLckLeft_B_Stat"
  BalrLeft_D_Stat/1 -> bus_creator/3  "BalrLeft_D_Stat"
  BalrMdeLeft_D_Stat/1 -> bus_creator/4  "BalrMdeLeft_D_Stat"
  BalrMdeSelLeft_B_Stat/1 -> bus_creator/5  "BalrMdeSelLeft_B_Stat"
  BalrSnsLeft_D_Falt/1 -> bus_creator/6  "BalrSnsLeft_D_Falt"
  BalrWndwLeft_B_Stat/1 -> bus_creator/7  "BalrWndwLeft_B_Stat"
  CamraRearOn_B_RqBalrl/1 -> bus_creator/8  "CamraRearOn_B_RqBalrl"
  DrLckActv_B_RqBalrl/1 -> bus_creator/9  "DrLckActv_B_RqBalrl"
  DrLckCnt_No_ActlBalrl/1 -> bus_creator/10  "DrLckCnt_No_ActlBalrl"
  WndwDrvRear_D_RqBalrl/1 -> bus_creator/11  "WndwDrvRear_D_RqBalrl"
  WndwDrv_D_RqBalrl/1 -> bus_creator/12  "WndwDrv_D_RqBalrl"
  WndwPsngrRear_D_RqBalrl/1 -> bus_creator/13  "WndwPsngrRear_D_RqBalrl"
  WndwPsngr_D_RqBalrl/1 -> bus_creator/14  "WndwPsngr_D_RqBalrl"

== system test_mdl/FD1_CAN_P702_GASD_MY21_DCV_V06/IPMA_ADAS/Bndry_Alert_R_Data ==
  BalrChimeRight_D_Rq : Constant
  BalrLckRight_B_Stat : Constant
  BalrMdeRight_D_Stat : Constant
  BalrMdeSelRight_B_Stat : Constant
  BalrRight_D_Stat : Constant
  BalrSnsRight_D_Falt : Constant
  BalrWndwRight_B_Stat : Constant
  CamraRearOn_B_RqBalrr : Constant
  DrLckActv_B_RqBalrr : Constant
  DrLckCnt_No_ActlBalrr : Constant
  WndwDrvRear_D_RqBalrr : Constant
  WndwDrv_D_RqBalrr : Constant
  WndwPsngrRear_D_RqBalrr : Constant
  WndwPsngr_D_RqBalrr : Constant
  bus_creator : BusCreator  Inputs=14
  port : Outport
  wires:
  bus_creator/1 -> port/1  "Bndry_Alert_R_Data"
  BalrChimeRight_D_Rq/1 -> bus_creator/1  "BalrChimeRight_D_Rq"
  BalrLckRight_B_Stat/1 -> bus_creator/2  "BalrLckRight_B_Stat"
  BalrMdeRight_D_Stat/1 -> bus_creator/3  "BalrMdeRight_D_Stat"
  BalrMdeSelRight_B_Stat/1 -> bus_creator/4  "BalrMdeSelRight_B_Stat"
  BalrRight_D_Stat/1 -> bus_creator/5  "BalrRight_D_Stat"
  BalrSnsRight_D_Falt/1 -> bus_creator/6  "BalrSnsRight_D_Falt"
  BalrWndwRight_B_Stat/1 -> bus_creator/7  "BalrWndwRight_B_Stat"
  CamraRearOn_B_RqBalrr/1 -> bus_creator/8  "CamraRearOn_B_RqBalrr"
  DrLckActv_B_RqBalrr/1 -> bus_creator/9  "DrLckActv_B_RqBalrr"
  DrLckCnt_No_ActlBalrr/1 -> bus_creator/10  "DrLckCnt_No_ActlBalrr"
  WndwDrvRear_D_RqBalrr/1 -> bus_creator/11  "WndwDrvRear_D_RqBalrr"
  WndwDrv_D_RqBalrr/1 -> bus_creator/12  "WndwDrv_D_RqBalrr"
  WndwPsngrRear_D_RqBalrr/1 -> bus_creator/13  "WndwPsngrRear_D_RqBalrr"
  WndwPsngr_D_RqBalrr/1 -> bus_creator/14  "WndwPsngr_D_RqBalrr"

== system test_mdl/FD1_CAN_P702_GASD_MY21_DCV_V06/IPMA_ADAS/BoundaryAlert_Left_1 ==
  BalrLeft1CurntX_L_Actl : Constant
  BalrLeft1CurntY_L_Actl : Constant
  BalrLeft1Dsply_B_Stat : Constant
  BalrLeft1Fast_B_Stat : Constant
  BalrLeft1Prev1X_L_Actl : Constant
  BalrLeft1Prev1Y_L_Actl : Constant
  BalrLeft1Prev2X_L_Actl : Constant
  BalrLeft1Prev2Y_L_Actl : Constant
  BalrLeft1Prev3X_L_Actl : Constant
  BalrLeft1Prev3Y_L_Actl : Constant
  BalrLeft1Threat_D_Stat : Constant
  bus_creator : BusCreator  Inputs=11
  port : Outport
  wires:
  bus_creator/1 -> port/1  "BoundaryAlert_Left_1"
  BalrLeft1CurntX_L_Actl/1 -> bus_creator/1  "BalrLeft1CurntX_L_Actl"
  BalrLeft1CurntY_L_Actl/1 -> bus_creator/2  "BalrLeft1CurntY_L_Actl"
  BalrLeft1Dsply_B_Stat/1 -> bus_creator/3  "BalrLeft1Dsply_B_Stat"
  BalrLeft1Fast_B_Stat/1 -> bus_creator/4  "BalrLeft1Fast_B_Stat"
  BalrLeft1Prev1X_L_Actl/1 -> bus_creator/5  "BalrLeft1Prev1X_L_Actl"
  BalrLeft1Prev1Y_L_Actl/1 -> bus_creator/6  "BalrLeft1Prev1Y_L_Actl"
  BalrLeft1Prev2X_L_Actl/1 -> bus_creator/7  "BalrLeft1Prev2X_L_Actl"
  BalrLeft1Prev2Y_L_Actl/1 -> bus_creator/8  "BalrLeft1Prev2Y_L_Actl"
  BalrLeft1Prev3X_L_Actl/1 -> bus_creator/9  "BalrLeft1Prev3X_L_Actl"
  BalrLeft1Prev3Y_L_Actl/1 -> bus_creator/10  "BalrLeft1Prev3Y_L_Actl"
  BalrLeft1Threat_D_Stat/1 -> bus_creator/11  "BalrLeft1Threat_D_Stat"

== system test_mdl/FD1_CAN_P702_GASD_MY21_DCV_V06/IPMA_ADAS/BoundaryAlert_Left_2 ==
  BalrLeft2CurntX_L_Actl : Constant
  BalrLeft2CurntY_L_Actl : Constant
  BalrLeft2Dsply_B_Stat : Constant
  BalrLeft2Fast_B_Stat : Constant
  BalrLeft2Prev1X_L_Actl : Constant
  BalrLeft2Prev1Y_L_Actl : Constant
  BalrLeft2Prev2X_L_Actl : Constant
  BalrLeft2Prev2Y_L_Actl : Constant
  BalrLeft2Prev3X_L_Actl : Constant
  BalrLeft2Prev3Y_L_Actl : Constant
  BalrLeft2Threat_D_Stat : Constant
  bus_creator : BusCreator  Inputs=11
  port : Outport
  wires:
  bus_creator/1 -> port/1  "BoundaryAlert_Left_2"
  BalrLeft2CurntX_L_Actl/1 -> bus_creator/1  "BalrLeft2CurntX_L_Actl"
  BalrLeft2CurntY_L_Actl/1 -> bus_creator/2  "BalrLeft2CurntY_L_Actl"
  BalrLeft2Dsply_B_Stat/1 -> bus_creator/3  "BalrLeft2Dsply_B_Stat"
  BalrLeft2Fast_B_Stat/1 -> bus_creator/4  "BalrLeft2Fast_B_Stat"
  BalrLeft2Prev1X_L_Actl/1 -> bus_creator/5  "BalrLeft2Prev1X_L_Actl"
  BalrLeft2Prev1Y_L_Actl/1 -> bus_creator/6  "BalrLeft2Prev1Y_L_Actl"
  BalrLeft2Prev2X_L_Actl/1 -> bus_creator/7  "BalrLeft2Prev2X_L_Actl"
  BalrLeft2Prev2Y_L_Actl/1 -> bus_creator/8  "BalrLeft2Prev2Y_L_Actl"
  BalrLeft2Prev3X_L_Actl/1 -> bus_creator/9  "BalrLeft2Prev3X_L_Actl"
  BalrLeft2Prev3Y_L_Actl/1 -> bus_creator/10  "BalrLeft2Prev3Y_L_Actl"
  BalrLeft2Threat_D_Stat/1 -> bus_creator/11  "BalrLeft2Threat_D_Stat"

== system test_mdl/FD1_CAN_P702_GASD_MY21_DCV_V06/IPMA_ADAS/BoundaryAlert_Left_3 ==
  BalrLeft3CurntX_L_Actl : Constant
  BalrLeft3CurntY_L_Actl : Constant
  BalrLeft3Dsply_B_Stat : Constant
  BalrLeft3Fast_B_Stat : Constant
  BalrLeft3Prev1X_L_Actl : Constant
  BalrLeft3Prev1Y_L_Actl : Constant
  BalrLeft3Prev2X_L_Actl : Constant
  BalrLeft3Prev2Y_L_Actl : Constant
  BalrLeft3Prev3X_L_Actl : Constant
  BalrLeft3Prev3Y_L_Actl : Constant
  BalrLeft3Threat_D_Stat : Constant
  bus_creator : BusCreator  Inputs=11
  port : Outport
  wires:
  bus_creator/1 -> port/1  "BoundaryAlert_Left_3"
  BalrLeft3CurntX_L_Actl/1 -> bus_creator/1  "BalrLeft3CurntX_L_Actl"
  BalrLeft3CurntY_L_Actl/1 -> bus_creator/2  "BalrLeft3CurntY_L_Actl"
  BalrLeft3Dsply_B_Stat/1 -> bus_creator/3  "BalrLeft3Dsply_B_Stat"
  BalrLeft3Fast_B_Stat/1 -> bus_creator/4  "BalrLeft3Fast_B_Stat"
  BalrLeft3Prev1X_L_Actl/1 -> bus_creator/5  "BalrLeft3Prev1X_L_Actl"
  BalrLeft3Prev1Y_L_Actl/1 -> bus_creator/6  "BalrLeft3Prev1Y_L_Actl"
  BalrLeft3Prev2X_L_Actl/1 -> bus_creator/7  "BalrLeft3Prev2X_L_Actl"
  BalrLeft3Prev2Y_L_Actl/1 -> bus_creator/8  "BalrLeft3Prev2Y_L_Actl"
  BalrLeft3Prev3X_L_Actl/1 -> bus_creator/9  "BalrLeft3Prev3X_L_Actl"
  BalrLeft3Prev3Y_L_Actl/1 -> bus_creator/10  "BalrLeft3Prev3Y_L_Actl"
  BalrLeft3Threat_D_Stat/1 -> bus_creator/11  "BalrLeft3Threat_D_Stat"

== system test_mdl/FD1_CAN_P702_GASD_MY21_DCV_V06/IPMA_ADAS/BoundaryAlert_Left_4 ==
  BalrLeft4CurntX_L_Actl : Constant
  BalrLeft4CurntY_L_Actl : Constant
  BalrLeft4Dsply_B_Stat : Constant
  BalrLeft4Fast_B_Stat : Constant
  BalrLeft4Prev1X_L_Actl : Constant
  BalrLeft4Prev1Y_L_Actl : Constant
  BalrLeft4Prev2X_L_Actl : Constant
  BalrLeft4Prev2Y_L_Actl : Constant
  BalrLeft4Prev3X_L_Actl : Constant
  BalrLeft4Prev3Y_L_Actl : Constant
  BalrLeft4Threat_D_Stat : Constant
  bus_creator : BusCreator  Inputs=11
  port : Outport
  wires:
  bus_creator/1 -> port/1  "BoundaryAlert_Left_4"
  BalrLeft4CurntX_L_Actl/1 -> bus_creator/1  "BalrLeft4CurntX_L_Actl"
  BalrLeft4CurntY_L_Actl/1 -> bus_creator/2  "BalrLeft4CurntY_L_Actl"
  BalrLeft4Dsply_B_Stat/1 -> bus_creator/3  "BalrLeft4Dsply_B_Stat"
  BalrLeft4Fast_B_Stat/1 -> bus_creator/4  "BalrLeft4Fast_B_Stat"
  BalrLeft4Prev1X_L_Actl/1 -> bus_creator/5  "BalrLeft4Prev1X_L_Actl"
  BalrLeft4Prev1Y_L_Actl/1 -> bus_creator/6  "BalrLeft4Prev1Y_L_Actl"
  BalrLeft4Prev2X_L_Actl/1 -> bus_creator/7  "BalrLeft4Prev2X_L_Actl"
  BalrLeft4Prev2Y_L_Actl/1 -> bus_creator/8  "BalrLeft4Prev2Y_L_Actl"
  BalrLeft4Prev3X_L_Actl/1 -> bus_creator/9  "BalrLeft4Prev3X_L_Actl"
  BalrLeft4Prev3Y_L_Actl/1 -> bus_creator/10  "BalrLeft4Prev3Y_L_Actl"
  BalrLeft4Threat_D_Stat/1 -> bus_creator/11  "BalrLeft4Threat_D_Stat"

== system test_mdl/FD1_CAN_P702_GASD_MY21_DCV_V06/IPMA_ADAS/BoundaryAlert_Right_1 ==
  BalrRight1CurntX_L_Actl : Constant
  BalrRight1CurntY_L_Actl : Constant
  BalrRight1Dsply_B_Stat : Constant
  BalrRight1Fast_B_Stat : Constant
  BalrRight1Prev1X_L_Actl : Constant
  BalrRight1Prev1Y_L_Actl : Constant
  BalrRight1Prev2X_L_Actl : Constant
  BalrRight1Prev2Y_L_Actl : Constant
  BalrRight1Prev3X_L_Actl : Constant
  BalrRight1Prev3Y_L_Actl : Constant
  BalrRight1Threat_D_Stat : Constant
  bus_creator : BusCreator  Inputs=11
  port : Outport
  wires:
  bus_creator/1 -> port/1  "BoundaryAlert_Right_1"
  BalrRight1CurntX_L_Actl/1 -> bus_creator/1  "BalrRight1CurntX_L_Actl"
  BalrRight1CurntY_L_Actl/1 -> bus_creator/2  "BalrRight1CurntY_L_Actl"
  BalrRight1Dsply_B_Stat/1 -> bus_creator/3  "BalrRight1Dsply_B_Stat"
  BalrRight1Fast_B_Stat/1 -> bus_creator/4  "BalrRight1Fast_B_Stat"
  BalrRight1Prev1X_L_Actl/1 -> bus_creator/5  "BalrRight1Prev1X_L_Actl"
  BalrRight1Prev1Y_L_Actl/1 -> bus_creator/6  "BalrRight1Prev1Y_L_Actl"
  BalrRight1Prev2X_L_Actl/1 -> bus_creator/7  "BalrRight1Prev2X_L_Actl"
  BalrRight1Prev2Y_L_Actl/1 -> bus_creator/8  "BalrRight1Prev2Y_L_Actl"
  BalrRight1Prev3X_L_Actl/1 -> bus_creator/9  "BalrRight1Prev3X_L_Actl"
  BalrRight1Prev3Y_L_Actl/1 -> bus_creator/10  "BalrRight1Prev3Y_L_Actl"
  BalrRight1Threat_D_Stat/1 -> bus_creator/11  "BalrRight1Threat_D_Stat"

== system test_mdl/FD1_CAN_P702_GASD_MY21_DCV_V06/IPMA_ADAS/BoundaryAlert_Right_2 ==
  BalrRight2CurntX_L_Actl : Constant
  BalrRight2CurntY_L_Actl : Constant
  BalrRight2Dsply_B_Stat : Constant
  BalrRight2Fast_B_Stat : Constant
  BalrRight2Prev1X_L_Actl : Constant
  BalrRight2Prev1Y_L_Actl : Constant
  BalrRight2Prev2X_L_Actl : Constant
  BalrRight2Prev2Y_L_Actl : Constant
  BalrRight2Prev3X_L_Actl : Constant
  BalrRight2Prev3Y_L_Actl : Constant
  BalrRight2Threat_D_Stat : Constant
  bus_creator : BusCreator  Inputs=11
  port : Outport
  wires:
  bus_creator/1 -> port/1  "BoundaryAlert_Right_2"
  BalrRight2CurntX_L_Actl/1 -> bus_creator/1  "BalrRight2CurntX_L_Actl"
  BalrRight2CurntY_L_Actl/1 -> bus_creator/2  "BalrRight2CurntY_L_Actl"
  BalrRight2Dsply_B_Stat/1 -> bus_creator/3  "BalrRight2Dsply_B_Stat"
  BalrRight2Fast_B_Stat/1 -> bus_creator/4  "BalrRight2Fast_B_Stat"
  BalrRight2Prev1X_L_Actl/1 -> bus_creator/5  "BalrRight2Prev1X_L_Actl"
  BalrRight2Prev1Y_L_Actl/1 -> bus_creator/6  "BalrRight2Prev1Y_L_Actl"
  BalrRight2Prev2X_L_Actl/1 -> bus_creator/7  "BalrRight2Prev2X_L_Actl"
  BalrRight2Prev2Y_L_Actl/1 -> bus_creator/8  "BalrRight2Prev2Y_L_Actl"
  BalrRight2Prev3X_L_Actl/1 -> bus_creator/9  "BalrRight2Prev3X_L_Actl"
  BalrRight2Prev3Y_L_Actl/1 -> bus_creator/10  "BalrRight2Prev3Y_L_Actl"
  BalrRight2Threat_D_Stat/1 -> bus_creator/11  "BalrRight2Threat_D_Stat"

== system test_mdl/FD1_CAN_P702_GASD_MY21_DCV_V06/IPMA_ADAS/BoundaryAlert_Right_3 ==
  BalrRight3CurntX_L_Actl : Constant
  BalrRight3CurntY_L_Actl : Constant
  BalrRight3Dsply_B_Stat : Constant
  BalrRight3Fast_B_Stat : Constant
  BalrRight3Prev1X_L_Actl : Constant
  BalrRight3Prev1Y_L_Actl : Constant
  BalrRight3Prev2X_L_Actl : Constant
  BalrRight3Prev2Y_L_Actl : Constant
  BalrRight3Prev3X_L_Actl : Constant
  BalrRight3Prev3Y_L_Actl : Constant
  BalrRight3Threat_D_Stat : Constant
  bus_creator : BusCreator  Inputs=11
  port : Outport
  wires:
  bus_creator/1 -> port/1  "BoundaryAlert_Right_3"
  BalrRight3CurntX_L_Actl/1 -> bus_creator/1  "BalrRight3CurntX_L_Actl"
  BalrRight3CurntY_L_Actl/1 -> bus_creator/2  "BalrRight3CurntY_L_Actl"
  BalrRight3Dsply_B_Stat/1 -> bus_creator/3  "BalrRight3Dsply_B_Stat"
  BalrRight3Fast_B_Stat/1 -> bus_creator/4  "BalrRight3Fast_B_Stat"
  BalrRight3Prev1X_L_Actl/1 -> bus_creator/5  "BalrRight3Prev1X_L_Actl"
  BalrRight3Prev1Y_L_Actl/1 -> bus_creator/6  "BalrRight3Prev1Y_L_Actl"
  BalrRight3Prev2X_L_Actl/1 -> bus_creator/7  "BalrRight3Prev2X_L_Actl"
  BalrRight3Prev2Y_L_Actl/1 -> bus_creator/8  "BalrRight3Prev2Y_L_Actl"
  BalrRight3Prev3X_L_Actl/1 -> bus_creator/9  "BalrRight3Prev3X_L_Actl"
  BalrRight3Prev3Y_L_Actl/1 -> bus_creator/10  "BalrRight3Prev3Y_L_Actl"
  BalrRight3Threat_D_Stat/1 -> bus_creator/11  "BalrRight3Threat_D_Stat"

== system test_mdl/FD1_CAN_P702_GASD_MY21_DCV_V06/IPMA_ADAS/BoundaryAlert_Right_4 ==
  BalrRight4CurntX_L_Actl : Constant
  BalrRight4CurntY_L_Actl : Constant
  BalrRight4Dsply_B_Stat : Constant
  BalrRight4Fast_B_Stat : Constant
  BalrRight4Prev1X_L_Actl : Constant
  BalrRight4Prev1Y_L_Actl : Constant
  BalrRight4Prev2X_L_Actl : Constant
  BalrRight4Prev2Y_L_Actl : Constant
  BalrRight4Prev3X_L_Actl : Constant
  BalrRight4Prev3Y_L_Actl : Constant
  BalrRight4Threat_D_Stat : Constant
  bus_creator : BusCreator  Inputs=11
  port : Outport
  wires:
  bus_creator/1 -> port/1  "BoundaryAlert_Right_4"
  BalrRight4CurntX_L_Actl/1 -> bus_creator/1  "BalrRight4CurntX_L_Actl"
  BalrRight4CurntY_L_Actl/1 -> bus_creator/2  "BalrRight4CurntY_L_Actl"
  BalrRight4Dsply_B_Stat/1 -> bus_creator/3  "BalrRight4Dsply_B_Stat"
  BalrRight4Fast_B_Stat/1 -> bus_creator/4  "BalrRight4Fast_B_Stat"
  BalrRight4Prev1X_L_Actl/1 -> bus_creator/5  "BalrRight4Prev1X_L_Actl"
  BalrRight4Prev1Y_L_Actl/1 -> bus_creator/6  "BalrRight4Prev1Y_L_Actl"
  BalrRight4Prev2X_L_Actl/1 -> bus_creator/7  "BalrRight4Prev2X_L_Actl"
  BalrRight4Prev2Y_L_Actl/1 -> bus_creator/8  "BalrRight4Prev2Y_L_Actl"
  BalrRight4Prev3X_L_Actl/1 -> bus_creator/9  "BalrRight4Prev3X_L_Actl"
  BalrRight4Prev3Y_L_Actl/1 -> bus_creator/10  "BalrRight4Prev3Y_L_Actl"
  BalrRight4Threat_D_Stat/1 -> bus_creator/11  "BalrRight4Threat_D_Stat"

== system test_mdl/FD1_CAN_P702_GASD_MY21_DCV_V06/IPMA_ADAS/GlareFreeBeam ==
  AdbBeam_D_Rq : Constant
  AdbBrdrBottom_An_Rq : Constant
  AdbBrdrLeft_An_Rq : Constant
  AdbBrdrLeft_L_Stat : Constant
  AdbBrdrRight_An_Rq : Constant
  AdbBrdrRight_L_Stat : Constant
  AdbBrdrTop_An_Rq : Constant
  AdbRamping_T_Rq : Constant
  bus_creator : BusCreator  Inputs=8
  port : Outport
  wires:
  bus_creator/1 -> port/1  "GlareFreeBeam"
  AdbBeam_D_Rq/1 -> bus_creator/1  "AdbBeam_D_Rq"
  AdbBrdrBottom_An_Rq/1 -> bus_creator/2  "AdbBrdrBottom_An_Rq"
  AdbBrdrLeft_An_Rq/1 -> bus_creator/3  "AdbBrdrLeft_An_Rq"
  AdbBrdrLeft_L_Stat/1 -> bus_creator/4  "AdbBrdrLeft_L_Stat"
  AdbBrdrRight_An_Rq/1 -> bus_creator/5  "AdbBrdrRight_An_Rq"
  AdbBrdrRight_L_Stat/1 -> bus_creator/6  "AdbBrdrRight_L_Stat"
  AdbBrdrTop_An_Rq/1 -> bus_creator/7  "AdbBrdrTop_An_Rq"
  AdbRamping_T_Rq/1 -> bus_creator/8  "AdbRamping_T_Rq"

== system test_mdl/FD1_CAN_P702_GASD_MY21_DCV_V06/IPMA_ADAS/IPMA_Data ==
  AhbHiBeam_D_Rq : Constant
  AhbcRampingV_D_Rq : Constant
  CamraDefog_B_Req : Constant
  CamraStats_D_Dsply : Constant
  DasAlrtLvl_D_Dsply : Constant
  DasStats_D_Dsply : Constant
  DasWarn_D_Dsply : Constant
  FeatConfigIpmaActl : Constant
  FeatNoIpmaActl : Constant
  LaActvStats_D_Dsply : Constant
  LaDenyStats_B_Dsply : Constant
  LaHandsOff_D_Dsply : Constant
  PersIndexIpma_D_Actl : Constant
  bus_creator : BusCreator  Inputs=13
  port : Outport
  wires:
  bus_creator/1 -> port/1  "IPMA_Data"
  AhbHiBeam_D_Rq/1 -> bus_creator/1  "AhbHiBeam_D_Rq"
  AhbcRampingV_D_Rq/1 -> bus_creator/2  "AhbcRampingV_D_Rq"
  CamraDefog_B_Req/1 -> bus_creator/3  "CamraDefog_B_Req"
  CamraStats_D_Dsply/1 -> bus_creator/4  "CamraStats_D_Dsply"
  DasAlrtLvl_D_Dsply/1 -> bus_creator/5  "DasAlrtLvl_D_Dsply"
  DasStats_D_Dsply/1 -> bus_creator/6  "DasStats_D_Dsply"
  DasWarn_D_Dsply/1 -> bus_creator/7  "DasWarn_D_Dsply"
  FeatConfigIpmaActl/1 -> bus_creator/8  "FeatConfigIpmaActl"
  FeatNoIpmaActl/1 -> bus_creator/9  "FeatNoIpmaActl"
  LaActvStats_D_Dsply/1 -> bus_creator/10  "LaActvStats_D_Dsply"
  LaDenyStats_B_Dsply/1 -> bus_creator/11  "LaDenyStats_B_Dsply"
  LaHandsOff_D_Dsply/1 -> bus_creator/12  "LaHandsOff_D_Dsply"
  PersIndexIpma_D_Actl/1 -> bus_creator/13  "PersIndexIpma_D_Actl"

== system test_mdl/FD1_CAN_P702_GASD_MY21_DCV_V06/IPMA_ADAS/IPMA_Data2 ==
  AdbDividedRoad_B_Stat : Constant
  AdbDrvSide_B_Stat : Constant
  DasAlrtInfo_D_Dsply : Constant
  IaccVLimUnit_D_Rq : Constant
  IaccVLim_D_Rq : Constant
  IsaVLimUnit_D_Rq : Constant
  IsaVLim_D_Rq : Constant
  LcwaMsgTxt_D_Stat : Constant
  LdwChime_B_Rq : Constant
  LongCtrlEnbl_D_Rq : Constant
  SblmPedCrossScnr_B_Stat : Constant
  SblmRndAbtScnr_B_Stat : Constant
  SblmStopScnr_B_Stat : Constant
  SblmYieldScnr_B_Stat : Constant
  TsrRegionTxt_D_Stat : Constant
  bus_creator : BusCreator  Inputs=15
  port : Outport
  wires:
  bus_creator/1 -> port/1  "IPMA_Data2"
  AdbDividedRoad_B_Stat/1 -> bus_creator/1  "AdbDividedRoad_B_Stat"
  AdbDrvSide_B_Stat/1 -> bus_creator/2  "AdbDrvSide_B_Stat"
  DasAlrtInfo_D_Dsply/1 -> bus_creator/3  "DasAlrtInfo_D_Dsply"
  IaccVLimUnit_D_Rq/1 -> bus_creator/4  "IaccVLimUnit_D_Rq"
  IaccVLim_D_Rq/1 -> bus_creator/5  "IaccVLim_D_Rq"
  IsaVLimUnit_D_Rq/1 -> bus_creator/6  "IsaVLimUnit_D_Rq"
  IsaVLim_D_Rq/1 -> bus_creator/7  "IsaVLim_D_Rq"
  LcwaMsgTxt_D_Stat/1 -> bus_creator/8  "LcwaMsgTxt_D_Stat"
  LdwChime_B_Rq/1 -> bus_creator/9  "LdwChime_B_Rq"
  LongCtrlEnbl_D_Rq/1 -> bus_creator/10  "LongCtrlEnbl_D_Rq"
  SblmPedCrossScnr_B_Stat/1 -> bus_creator/11  "SblmPedCrossScnr_B_Stat"
  SblmRndAbtScnr_B_Stat/1 -> bus_creator/12  "SblmRndAbtScnr_B_Stat"
  SblmStopScnr_B_Stat/1 -> bus_creator/13  "SblmStopScnr_B_Stat"
  SblmYieldScnr_B_Stat/1 -> bus_creator/14  "SblmYieldScnr_B_Stat"
  TsrRegionTxt_D_Stat/1 -> bus_creator/15  "TsrRegionTxt_D_Stat"

== system test_mdl/FD1_CAN_P702_GASD_MY21_DCV_V06/IPMA_ADAS/IPMA_Data3 ==
  AdbUrbanArea_B_Stat : Constant
  CbdblActv_B_RqAdas : Constant
  LightCurv_NoRate_Actl : Constant
  LightCurv_No_Actl : Constant
  LightPathOffst_L_Actl : Constant
  LightPath_An_Actl : Constant
  LightRng_L_Max : Constant
  MbdblActv_B_RqAdas : Constant
  bus_creator : BusCreator  Inputs=8
  port : Outport
  wires:
  bus_creator/1 -> port/1  "IPMA_Data3"
  AdbUrbanArea_B_Stat/1 -> bus_creator/1  "AdbUrbanArea_B_Stat"
  CbdblActv_B_RqAdas/1 -> bus_creator/2  "CbdblActv_B_RqAdas"
  LightCurv_NoRate_Actl/1 -> bus_creator/3  "LightCurv_NoRate_Actl"
  LightCurv_No_Actl/1 -> bus_creator/4  "LightCurv_No_Actl"
  LightPathOffst_L_Actl/1 -> bus_creator/5  "LightPathOffst_L_Actl"
  LightPath_An_Actl/1 -> bus_creator/6  "LightPath_An_Actl"
  LightRng_L_Max/1 -> bus_creator/7  "LightRng_L_Max"
  MbdblActv_B_RqAdas/1 -> bus_creator/8  "MbdblActv_B_RqAdas"

== system test_mdl/FD1_CAN_P702_GASD_MY21_DCV_V06/IPMA_ADAS/IPMA_Data4 ==
  AdasLcDistToObj_L_Actl : Constant
  VehVActlAdas_D_Qf : Constant
  Veh_V_ActlAdas : Constant
  Veh_V_RqLsc : Constant
  bus_creator : BusCreator  Inputs=4
  port : Outport
  wires:
  bus_creator/1 -> port/1  "IPMA_Data4"
  AdasLcDistToObj_L_Actl/1 -> bus_creator/1  "AdasLcDistToObj_L_Actl"
  VehVActlAdas_D_Qf/1 -> bus_creator/2  "VehVActlAdas_D_Qf"
  Veh_V_ActlAdas/1 -> bus_creator/3  "Veh_V_ActlAdas"
  Veh_V_RqLsc/1 -> bus_creator/4  "Veh_V_RqLsc"

== system test_mdl/FD1_CAN_P702_GASD_MY21_DCV_V06/IPMA_ADAS/Image_Processing_Data ==
  BrkDecel_B_RqRba : Constant
  BrkEnbl_B_RqRba : Constant
  CamraFrntStat_D_Stat : Constant
  RbaAlrt_D_Dsply : Constant
  RbaMnu_D_Rq : Constant
  RbaMsg_D_Rq : Constant
  Rba_D_Stat : Constant
  TrlrAidEnbl_D_RqAdas : Constant
  TrlrAidSwtchLamp_B_Rq : Constant
  TrlrHitchChime_D_Rq : Constant
  TrlrHitchIcon_D_Rq : Constant
  TrlrHitchLamp_D_Rq2 : Constant
  TrlrHitchMsgTxt_D_Rq : Constant
  TrlrRvrseEnbl_D2_Stat : Constant
  TrlrRvrseMsgTxt_D2_Rq : Constant
  bus_creator : BusCreator  Inputs=15
  port : Outport
  wires:
  bus_creator/1 -> port/1  "Image_Processing_Data"
  BrkDecel_B_RqRba/1 -> bus_creator/1  "BrkDecel_B_RqRba"
  BrkEnbl_B_RqRba/1 -> bus_creator/2  "BrkEnbl_B_RqRba"
  CamraFrntStat_D_Stat/1 -> bus_creator/3  "CamraFrntStat_D_Stat"
  RbaAlrt_D_Dsply/1 -> bus_creator/4  "RbaAlrt_D_Dsply"
  RbaMnu_D_Rq/1 -> bus_creator/5  "RbaMnu_D_Rq"
  RbaMsg_D_Rq/1 -> bus_creator/6  "RbaMsg_D_Rq"
  Rba_D_Stat/1 -> bus_creator/7  "Rba_D_Stat"
  TrlrAidEnbl_D_RqAdas/1 -> bus_creator/8  "TrlrAidEnbl_D_RqAdas"
  TrlrAidSwtchLamp_B_Rq/1 -> bus_creator/9  "TrlrAidSwtchLamp_B_Rq"
  TrlrHitchChime_D_Rq/1 -> bus_creator/10  "TrlrHitchChime_D_Rq"
  TrlrHitchIcon_D_Rq/1 -> bus_creator/11  "TrlrHitchIcon_D_Rq"
  TrlrHitchLamp_D_Rq2/1 -> bus_creator/12  "TrlrHitchLamp_D_Rq2"
  TrlrHitchMsgTxt_D_Rq/1 -> bus_creator/13  "TrlrHitchMsgTxt_D_Rq"
  TrlrRvrseEnbl_D2_Stat/1 -> bus_creator/14  "TrlrRvrseEnbl_D2_Stat"
  TrlrRvrseMsgTxt_D2_Rq/1 -> bus_creator/15  "TrlrRvrseMsgTxt_D2_Rq"

== system test_mdl/FD1_CAN_P702_GASD_MY21_DCV_V06/IPMA_ADAS/Lane_Assist_Data1 ==
  LaCurvature_No_Calc : Constant
  LaRampType_B_Req : Constant
  LaRefAng_No_Req : Constant
  LdwActvIntns_D_Req : Constant
  LdwActvStats_D_Req : Constant
  LkaActvStats_D2_Req : Constant
  LkaDrvOvrrd_D_Rq : Constant
  bus_creator : BusCreator  Inputs=7
  port : Outport
  wires:
  bus_creator/1 -> port/1  "Lane_Assist_Data1"
  LaCurvature_No_Calc/1 -> bus_creator/1  "LaCurvature_No_Calc"
  LaRampType_B_Req/1 -> bus_creator/2  "LaRampType_B_Req"
  LaRefAng_No_Req/1 -> bus_creator/3  "LaRefAng_No_Req"
  LdwActvIntns_D_Req/1 -> bus_creator/4  "LdwActvIntns_D_Req"
  LdwActvStats_D_Req/1 -> bus_creator/5  "LdwActvStats_D_Req"
  LkaActvStats_D2_Req/1 -> bus_creator/6  "LkaActvStats_D2_Req"
  LkaDrvOvrrd_D_Rq/1 -> bus_creator/7  "LkaDrvOvrrd_D_Rq"

== system test_mdl/FD1_CAN_P702_GASD_MY21_DCV_V06/IPMA_ADAS/LateralMotionControl ==
  HandsOffCnfm_B_Rq : Constant
  LatCtlCurv_NoRate_Actl : Constant
  LatCtlCurv_No_Actl : Constant
  LatCtlPathOffst_L_Actl : Constant
  LatCtlPath_An_Actl : Constant
  LatCtlPrecision_D_Rq : Constant
  LatCtlRampType_D_Rq : Constant
  LatCtlRng_L_Max : Constant
  LatCtl_D_Rq : Constant
  bus_creator : BusCreator  Inputs=9
  port : Outport
  wires:
  bus_creator/1 -> port/1  "LateralMotionControl"
  HandsOffCnfm_B_Rq/1 -> bus_creator/1  "HandsOffCnfm_B_Rq"
  LatCtlCurv_NoRate_Actl/1 -> bus_creator/2  "LatCtlCurv_NoRate_Actl"
  LatCtlCurv_No_Actl/1 -> bus_creator/3  "LatCtlCurv_No_Actl"
  LatCtlPathOffst_L_Actl/1 -> bus_creator/4  "LatCtlPathOffst_L_Actl"
  LatCtlPath_An_Actl/1 -> bus_creator/5  "LatCtlPath_An_Actl"
  LatCtlPrecision_D_Rq/1 -> bus_creator/6  "LatCtlPrecision_D_Rq"
  LatCtlRampType_D_Rq/1 -> bus_creator/7  "LatCtlRampType_D_Rq"
  LatCtlRng_L_Max/1 -> bus_creator/8  "LatCtlRng_L_Max"
  LatCtl_D_Rq/1 -> bus_creator/9  "LatCtl_D_Rq"

== system test_mdl/FD1_CAN_P702_GASD_MY21_DCV_V06/IPMA_ADAS/LateralMotionControl2 ==
  HandsOffCnfm_B_Rq : Constant
  LatCtlCrv_NoRate2_Actl : Constant
  LatCtlCurv_No_Actl : Constant
  LatCtlPathOffst_L_Actl : Constant
  LatCtlPath_An_Actl : Constant
  LatCtlPath_No_Cnt : Constant
  LatCtlPath_No_Cs : Constant
  LatCtlPrecision_D_Rq : Constant
  LatCtlRampType_D_Rq : Constant
  LatCtl_D2_Rq : Constant
  bus_creator : BusCreator  Inputs=10
  port : Outport
  wires:
  bus_creator/1 -> port/1  "LateralMotionControl2"
  HandsOffCnfm_B_Rq/1 -> bus_creator/1  "HandsOffCnfm_B_Rq"
  LatCtlCrv_NoRate2_Actl/1 -> bus_creator/2  "LatCtlCrv_NoRate2_Actl"
  LatCtlCurv_No_Actl/1 -> bus_creator/3  "LatCtlCurv_No_Actl"
  LatCtlPathOffst_L_Actl/1 -> bus_creator/4  "LatCtlPathOffst_L_Actl"
  LatCtlPath_An_Actl/1 -> bus_creator/5  "LatCtlPath_An_Actl"
  LatCtlPath_No_Cnt/1 -> bus_creator/6  "LatCtlPath_No_Cnt"
  LatCtlPath_No_Cs/1 -> bus_creator/7  "LatCtlPath_No_Cs"
  LatCtlPrecision_D_Rq/1 -> bus_creator/8  "LatCtlPrecision_D_Rq"
  LatCtlRampType_D_Rq/1 -> bus_creator/9  "LatCtlRampType_D_Rq"
  LatCtl_D2_Rq/1 -> bus_creator/10  "LatCtl_D2_Rq"

== system test_mdl/FD1_CAN_P702_GASD_MY21_DCV_V06/IPMA_ADAS/OTAPhysCCMtoGWM_ECG ==
  OTAPhysCCMtoGWM_ECG : Constant
  bus_creator : BusCreator  Inputs=1
  port : Outport
  wires:
  bus_creator/1 -> port/1  "OTAPhysCCMtoGWM_ECG"
  OTAPhysCCMtoGWM_ECG/1 -> bus_creator/1  "OTAPhysCCMtoGWM_ECG"

== system test_mdl/FD1_CAN_P702_GASD_MY21_DCV_V06/IPMA_ADAS/OTAPhysIPMAtoGWM_ECG ==
  OTAPhysIPMAtoGWM_ECG : Constant
  bus_creator : BusCreator  Inputs=1
  port : Outport
  wires:
  bus_creator/1 -> port/1  "OTAPhysIPMAtoGWM_ECG"
  OTAPhysIPMAtoGWM_ECG/1 -> bus_creator/1  "OTAPhysIPMAtoGWM_ECG"

== system test_mdl/FD1_CAN_P702_GASD_MY21_DCV_V06/IPMA_ADAS/OTAPhysSODCMCtoGWM_ECG ==
  OTAPhysSODCMCtoGWM_ECG : Constant
  bus_creator : BusCreator  Inputs=1
  port : Outport
  wires:
  bus_creator/1 -> port/1  "OTAPhysSODCMCtoGWM_ECG"
  OTAPhysSODCMCtoGWM_ECG/1 -> bus_creator/1  "OTAPhysSODCMCtoGWM_ECG"

== system test_mdl/FD1_CAN_P702_GASD_MY21_DCV_V06/IPMA_ADAS/OTAPhysSODCMDtoGWM_ECG ==
  OTAPhysSODCMDtoGWM_ECG : Constant
  bus_creator : BusCreator  Inputs=1
  port : Outport
  wires:
  bus_creator/1 -> port/1  "OTAPhysSODCMDtoGWM_ECG"
  OTAPhysSODCMDtoGWM_ECG/1 -> bus_creator/1  "OTAPhysSODCMDtoGWM_ECG"

== system test_mdl/FD1_CAN_P702_GASD_MY21_DCV_V06/IPMA_ADAS/OTAPhysSODLtoGWM_ECG ==
  OTAPhysSODLtoGWM_ECG : Constant
  bus_creator : BusCreator  Inputs=1
  port : Outport
  wires:
  bus_creator/1 -> port/1  "OTAPhysSODLtoGWM_ECG"
  OTAPhysSODLtoGWM_ECG/1 -> bus_creator/1  "OTAPhysSODLtoGWM_ECG"

== system test_mdl/FD1_CAN_P702_GASD_MY21_DCV_V06/IPMA_ADAS/OTAPhysSODRtoGWM_ECG ==
  OTAPhysSODRtoGWM_ECG : Constant
  bus_creator : BusCreator  Inputs=1
  port : Outport
  wires:
  bus_creator/1 -> port/1  "OTAPhysSODRtoGWM_ECG"
  OTAPhysSODRtoGWM_ECG/1 -> bus_creator/1  "OTAPhysSODRtoGWM_ECG"

== system test_mdl/FD1_CAN_P702_GASD_MY21_DCV_V06/IPMA_ADAS/PARSEDPhysCCMtoGWM_ECG ==
  PARSEDPhysCCMtoGWM_ECG : Constant
  bus_creator : BusCreator  Inputs=1
  port : Outport
  wires:
  bus_creator/1 -> port/1  "PARSEDPhysCCMtoGWM_ECG"
  PARSEDPhysCCMtoGWM_ECG/1 -> bus_creator/1  "PARSEDPhysCCMtoGWM_ECG"

== system test_mdl/FD1_CAN_P702_GASD_MY21_DCV_V06/IPMA_ADAS/PARSEDPhysIPMAtoGWM_ECG ==
  PARSEDPhysIPMAtoGWM_ECG : Constant
  bus_creator : BusCreator  Inputs=1
  port : Outport
  wires:
  bus_creator/1 -> port/1  "PARSEDPhysIPMAtoGWM_ECG"
  PARSEDPhysIPMAtoGWM_ECG/1 -> bus_creator/1  "PARSEDPhysIPMAtoGWM_ECG"

== system test_mdl/FD1_CAN_P702_GASD_MY21_DCV_V06/IPMA_ADAS/PARSEDPhysSODCMCtoGWM_ECG ==
  PARSEDPhysSODCMCtoGWM_ECG : Constant
  bus_creator : BusCreator  Inputs=1
  port : Outport
  wires:
  bus_creator/1 -> port/1  "PARSEDPhysSODCMCtoGWM_ECG"
  PARSEDPhysSODCMCtoGWM_ECG/1 -> bus_creator/1  "PARSEDPhysSODCMCtoGWM_ECG"

== system test_mdl/FD1_CAN_P702_GASD_MY21_DCV_V06/IPMA_ADAS/PARSEDPhysSODCMDtoGWM_ECG ==
  PARSEDPhysSODCMDtoGWM_ECG : Constant
  bus_creator : BusCreator  Inputs=1
  port : Outport
  wires:
  bus_creator/1 -> port/1  "PARSEDPhysSODCMDtoGWM_ECG"
  PARSEDPhysSODCMDtoGWM_ECG/1 -> bus_creator/1  "PARSEDPhysSODCMDtoGWM_ECG"
